simulink model "s7segm_top"  (R2023a)
settings: Solver=VariableStepAuto  StartTime=0.0  StopTime=2  RelTol=1e-3
libraries: simulink x11, hdlsllib x1
settings Model: Creator=criedl  LastModifiedBy=eduyilmet001
settings OptimizationCC: BlockReduction=off  ConditionallyExecuteInputs=off
settings DebuggingCC: UnconnectedInputMsg=warning  UnconnectedOutputMsg=warning  UnconnectedLineMsg=warning
settings ModelReferenceCC: EnableRefExpFcnMdlSchedulingChecks=on
settings RTWCC: DLArmComputeVersion=19.05

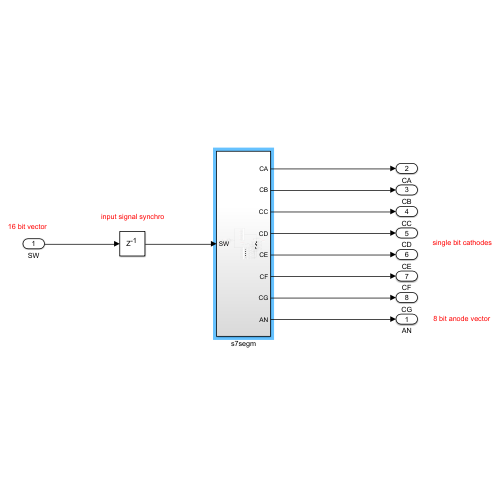
[thumbnail: Simulink's stored preview of the top-level diagram]
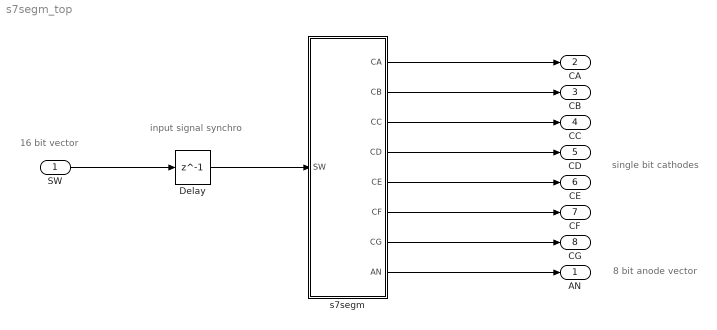
== system s7segm_top ==
  note: input signal synchro
  note: 16 bit vector
  note: 8 bit anode vector
  note: single bit cathodes
  SW : Inport  OutDataTypeStr=fixdt(0,16,0)
  Delay : Delay  DelayLength=1  InitialCondition=0
  s7segm : Subsystem
  AN : Outport  InitialOutput=0
  CA : Outport  Port=2  InitialOutput=0
  CB : Outport  Port=3  InitialOutput=0
  CC : Outport  Port=4  InitialOutput=0
  CD : Outport  Port=5  InitialOutput=0
  CE : Outport  Port=6  InitialOutput=0
  CF : Outport  Port=7  InitialOutput=0
  CG : Outport  Port=8  InitialOutput=0
  wires:
  s7segm/6(CF) -> CF/1
  s7segm/5(CE) -> CE/1
  s7segm/7(CG) -> CG/1
  s7segm/1(CA) -> CA/1
  s7segm/3(CC) -> CC/1
  s7segm/4(CD) -> CD/1
  s7segm/2(CB) -> CB/1
  SW/1 -> Delay/1
  Delay/1 -> s7segm/1(SW)
  s7segm/8(AN) -> AN/1

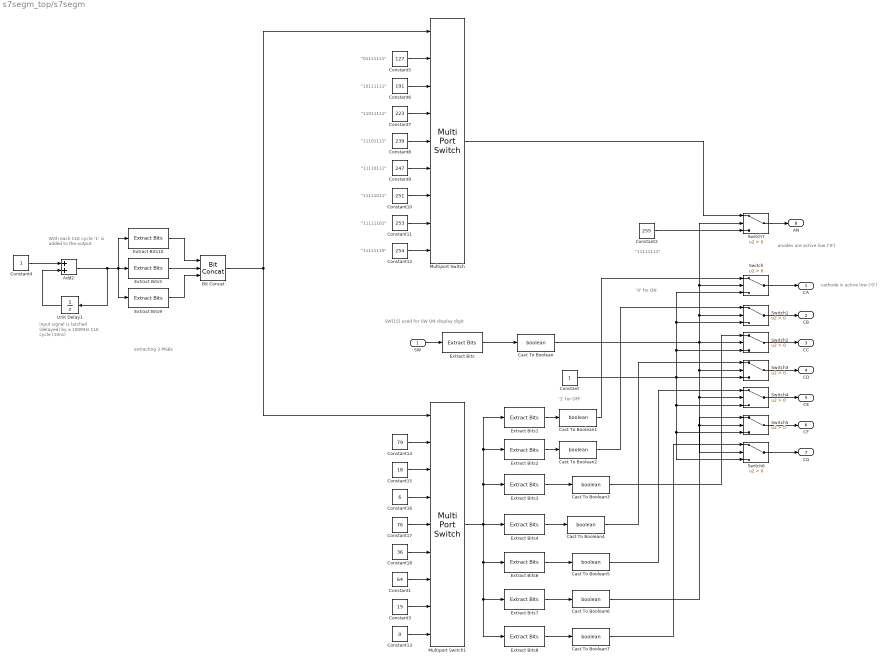
== system s7segm_top/s7segm ==
  note: cathode is active low ('0')
  note: SW(15) used for SW ON display digit
  note: '0' for ON
  note: "01111111"
  note: "11111111"
  note: '1' for OFF
  note: anodes are active low ('0')
  note: With each CLK cycle '1' is added to the output
  note: input signal is latched (delayed) by a 100MHz CLK cycle (10ns)
  note: extracting 3 MSBs
  note: "10111111"
  note: "11011111"
  note: "11101111"
  note: "11110111"
  note: "11111011"
  note: "11111101"
  note: "11111110"
  SW : Inport
  Add2 : Sum  AccumDataTypeStr=fixdt(0,20,0)  OutDataTypeStr=fixdt(0,20,0)
  Bit Concat : hdlsllib/Logic and Bit Operations/Bit Concat  numInputs=3
  Cast To Boolean{,1..7} (8 alike) : DataTypeConversion  OutDataTypeStr=boolean  SaturateOnIntegerOverflow=off  RndMeth=Floor
  Constant : Constant  OutDataTypeStr=boolean
  Constant1 : Constant  Value=64  OutDataTypeStr=fixdt(0,8,0)
  Constant10 : Constant  Value=251  OutDataTypeStr=uint8
  Constant11 : Constant  Value=253  OutDataTypeStr=uint8
  Constant12 : Constant  Value=254  OutDataTypeStr=uint8
  Constant13 : Constant  Value=0  OutDataTypeStr=fixdt(0,8,0)
  Constant14 : Constant  Value=79  OutDataTypeStr=fixdt(0,8,0)
  Constant15 : Constant  Value=18  OutDataTypeStr=fixdt(0,8,0)
  Constant16 : Constant  Value=6  OutDataTypeStr=fixdt(0,8,0)
  Constant17 : Constant  Value=76  OutDataTypeStr=fixdt(0,8,0)
  Constant18 : Constant  Value=36  OutDataTypeStr=fixdt(0,8,0)
  Constant2 : Constant  Value=255  OutDataTypeStr=fixdt(0,8,0)
  Constant3 : Constant  Value=15  OutDataTypeStr=fixdt(0,8,0)
  Constant4 : Constant  OutDataTypeStr=boolean
  Constant5 : Constant  Value=127  OutDataTypeStr=uint8
  Constant6 : Constant  Value=191  OutDataTypeStr=uint8
  Constant7 : Constant  Value=223  OutDataTypeStr=uint8
  Constant8 : Constant  Value=239  OutDataTypeStr=uint8
  Constant9 : Constant  Value=247  OutDataTypeStr=uint8
  Extract Bits : simulink/Logic and Bit Operations/Extract Bits  bitsToExtract=Range of bits  numBits=8  bitIdxRange=[15 15]  outScalingMode=Preserve fixed-point scaling
  Extract Bits1 : simulink/Logic and Bit Operations/Extract Bits  bitsToExtract=Range of bits  numBits=8  bitIdxRange=[6 6]  outScalingMode=Preserve fixed-point scaling
  Extract Bits10 : simulink/Logic and Bit Operations/Extract Bits  bitsToExtract=Range of bits  numBits=8  bitIdxRange=[19 19]  outScalingMode=Preserve fixed-point scaling
  Extract Bits2 : simulink/Logic and Bit Operations/Extract Bits  bitsToExtract=Range of bits  numBits=8  bitIdxRange=[5 5]  outScalingMode=Preserve fixed-point scaling
  Extract Bits3 : simulink/Logic and Bit Operations/Extract Bits  bitsToExtract=Range of bits  numBits=8  bitIdxRange=[4 4]  outScalingMode=Preserve fixed-point scaling
  Extract Bits4 : simulink/Logic and Bit Operations/Extract Bits  bitsToExtract=Range of bits  numBits=8  bitIdxRange=[3 3]  outScalingMode=Preserve fixed-point scaling
  Extract Bits5 : simulink/Logic and Bit Operations/Extract Bits  bitsToExtract=Range of bits  numBits=8  bitIdxRange=[18 18]  outScalingMode=Preserve fixed-point scaling
  Extract Bits6 : simulink/Logic and Bit Operations/Extract Bits  bitsToExtract=Range of bits  numBits=8  bitIdxRange=[2 2]  outScalingMode=Preserve fixed-point scaling
  Extract Bits7 : simulink/Logic and Bit Operations/Extract Bits  bitsToExtract=Range of bits  numBits=8  bitIdxRange=[1 1]  outScalingMode=Preserve fixed-point scaling
  Extract Bits8 : simulink/Logic and Bit Operations/Extract Bits  bitsToExtract=Range of bits  numBits=8  bitIdxRange=[0 0]  outScalingMode=Preserve fixed-point scaling
  Extract Bits9 : simulink/Logic and Bit Operations/Extract Bits  bitsToExtract=Range of bits  numBits=8  bitIdxRange=[17 17]  outScalingMode=Preserve fixed-point scaling
  Multiport Switch : MultiPortSwitch  Inputs=8  OutDataTypeStr=fixdt(0,8,0)  SaturateOnIntegerOverflow=off  InputSameDT=off
  Multiport Switch1 : MultiPortSwitch  Inputs=8  OutDataTypeStr=fixdt(0,8,0)  SaturateOnIntegerOverflow=off  InputSameDT=off
  Switch{,1..7} (8 alike) : Switch  Criteria=u2 > Threshold  SaturateOnIntegerOverflow=off  InputSameDT=off
  Unit Delay1 : UnitDelay  SampleTime=-1  HasFrameUpgradeWarning=on
  CA : Outport
  CB : Outport  Port=2
  CC : Outport  Port=3
  CD : Outport  Port=4
  CE : Outport  Port=5
  CF : Outport  Port=6
  CG : Outport  Port=7
  AN : Outport  Port=8
  wires:
  Constant2/1 -> Switch7/3
  Constant/1 -> Switch/3, Switch1/3, Switch2/3, Switch3/3, Switch4/3, Switch5/3, Switch6/3
  Cast To Boolean/1 -> Switch6/2, Switch5/2, Switch4/2, Switch3/2, Switch2/2, Switch1/2, Switch/2, Switch7/2
  Switch3/1 -> CD/1
  Switch6/1 -> CG/1
  Extract Bits/1 -> Cast To Boolean/1
  Switch/1 -> CA/1
  Switch4/1 -> CE/1
  Switch2/1 -> CC/1
  Switch1/1 -> CB/1
  Switch5/1 -> CF/1
  SW/1 -> Extract Bits/1
  Add2/1 -> Extract Bits9/1, Extract Bits10/1, Extract Bits5/1, Unit Delay1/1
  Unit Delay1/1 -> Add2/2
  Constant4/1 -> Add2/1
  Constant12/1 -> Multiport Switch/9
  Constant11/1 -> Multiport Switch/8
  Constant10/1 -> Multiport Switch/7
  Constant9/1 -> Multiport Switch/6
  Constant8/1 -> Multiport Switch/5
  Constant7/1 -> Multiport Switch/4
  Constant6/1 -> Multiport Switch/3
  Constant5/1 -> Multiport Switch/2
  Switch7/1 -> AN/1
  Multiport Switch/1 -> Switch7/1
  Constant14/1 -> Multiport Switch1/2
  Constant16/1 -> Multiport Switch1/4
  Constant15/1 -> Multiport Switch1/3
  Constant17/1 -> Multiport Switch1/5
  Constant18/1 -> Multiport Switch1/6
  Constant1/1 -> Multiport Switch1/7
  Constant3/1 -> Multiport Switch1/8
  Constant13/1 -> Multiport Switch1/9
  Multiport Switch1/1 -> Extract Bits1/1, Extract Bits2/1, Extract Bits3/1, Extract Bits7/1, Extract Bits8/1, Extract Bits6/1, Extract Bits4/1
  Extract Bits1/1 -> Cast To Boolean1/1
  Extract Bits2/1 -> Cast To Boolean2/1
  Extract Bits3/1 -> Cast To Boolean3/1
  Extract Bits4/1 -> Cast To Boolean4/1
  Extract Bits6/1 -> Cast To Boolean5/1
  Extract Bits7/1 -> Cast To Boolean6/1
  Extract Bits8/1 -> Cast To Boolean7/1
  Extract Bits5/1 -> Bit Concat/2
  Extract Bits10/1 -> Bit Concat/1
  Extract Bits9/1 -> Bit Concat/3
  Bit Concat/1 -> Multiport Switch/1, Multiport Switch1/1
  Cast To Boolean1/1 -> Switch/1
  Cast To Boolean2/1 -> Switch1/1
  Cast To Boolean3/1 -> Switch2/1
  Cast To Boolean4/1 -> Switch3/1
  Cast To Boolean5/1 -> Switch4/1
  Cast To Boolean6/1 -> Switch5/1
  Cast To Boolean7/1 -> Switch6/1
